simulink model "RL_Vdc_thy"  (R2020b)
settings: Solver=VariableStepAuto  StartTime=0.0  StopTime=0.02  RelTol=1e-3
undefined symbols (not defined in the file): Angle, Magnitude
libraries: powerlib x13, powerlib_meascontrol x3
settings Model: Creator=SAN  LastModifiedBy=macbook
settings DataIOCC: ReturnWorkspaceOutputs=off
settings DebuggingCC: ArithmeticOperatorsInVariantConditions=warning
settings SFSimCC: SimUseLocalCustomCode=off  CustomCodeUndefinedFunction=UseInterfaceOnly
settings RTWCC: RTWUseLocalCustomCode=off

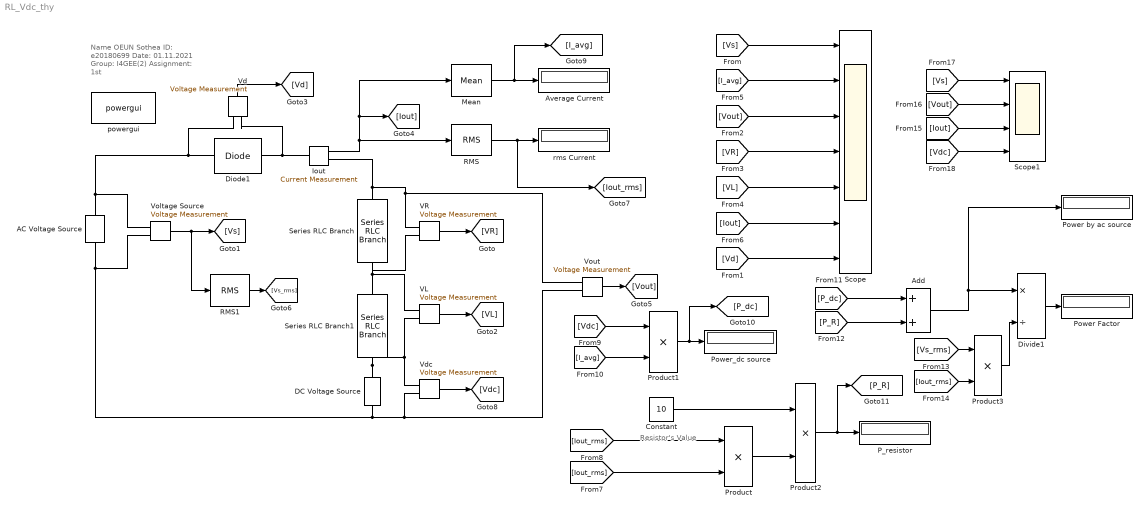
== system RL_Vdc_thy ==
  note: Resistor's Value
  note: Name OEUN Sothea
      | ID: e20180699
      | Date: 01.11.2021
      | Group: I4GEE(2)
      | Assignment: 1st
  " Power by ac source " : Display
  AC Voltage Source : powerlib/Electrical Sources/AC Voltage Source  Amplitude=120*sqrt(2)  Phase=0  Frequency=60  SampleTime=0  Measurements=None  BusType=swing  Pref=10e3  Qref=0  Qmin=-inf  Qmax=+inf
  Add : Sum
  Average Current : Display
  Constant : Constant  Value=10  SampleTime=0
  DC Voltage Source : powerlib/Electrical Sources/DC Voltage Source  Amplitude=100  Measurements=None
  Diode1 : powerlib/Power Electronics/Diode  Ron=0.001  Lon=0  Vf=0.8  IC=0  UseSnubber=0  Rs=500  Cs=250e-9  Measurements=off
  Divide1 : Product  Inputs=*/
  Iout : powerlib/Measurements/Current Measurement  PhasorSimulation=off  OutputType=Magnitude  PSBequivalent=0
  Mean : powerlib_meascontrol/Measurements/Mean  Freq=60  Vinit=0  Ts=0
  P_resistor : Display
  "Power Factor " : Display
  Power_dc source : Display
  Product{,1..3} (4 alike) : Product
  RMS : powerlib_meascontrol/Measurements/RMS  TrueRMS=on  Freq=60  RMSInit=120  Ts=0
  RMS1 : powerlib_meascontrol/Measurements/RMS  TrueRMS=on  Freq=60  RMSInit=120  Ts=0
  Scope : Scope  NumInputPorts=7
  Scope1 : Scope  NumInputPorts=4
  Series RLC Branch : powerlib/Elements/Series RLC Branch  LConnTagsString=__new0  RConnTagsString=__new0  BranchType=R  Resistance=10  Inductance=0.1  SetiL0=off  InitialCurrent=0  Capacitance=1e-6  Setx0=off  InitialVoltage=0  Measurements=None
  Series RLC Branch1 : powerlib/Elements/Series RLC Branch  LConnTagsString=__new0  RConnTagsString=__new0  BranchType=L  Resistance=100  Inductance=0.075  SetiL0=off  InitialCurrent=0  Capacitance=1e-6  Setx0=off  InitialVoltage=0  Measurements=None
  VL : powerlib/Measurements/Voltage Measurement  PhasorSimulation=off  OutputType=Magnitude-Angle  PSBequivalent=0
  "VR " : powerlib/Measurements/Voltage Measurement  PhasorSimulation=off  OutputType=Complex  PSBequivalent=0
  Vd : powerlib/Measurements/Voltage Measurement  PhasorSimulation=off  OutputType=Complex  PSBequivalent=0
  Vdc : powerlib/Measurements/Voltage Measurement  PhasorSimulation=off  OutputType=Magnitude-Angle  PSBequivalent=0
  "Voltage Source " : powerlib/Measurements/Voltage Measurement  PhasorSimulation=off  OutputType=Complex  PSBequivalent=0
  "Vout " : powerlib/Measurements/Voltage Measurement  PhasorSimulation=off  OutputType=Magnitude-Angle  PSBequivalent=0
  powergui : powerlib/powergui  Priority=1  SimulationMode=Continuous  SampleTime=50e-6  frequency=60  Iterations=50  frequencyindice=60  Pbase=100e6  ErrMax=1e-4  UnitsV=kV  UnitsW=MW  buscounter=0  FunctionMessages=off  echomessages=off  EnableUseOfTLC=off  CurrentSourceSwitches=off  DisableSnubberDevices=off  DisableRonSwitches=off  DisableVfSwitches=off  DisplayEquations=off  AutomaticDiscreteSolvers=off  SolverType=Tustin/Backward Euler (TBE)  Interpol=off  ExternalGateDelay=off  methode=off  Ts=100  x0status=blocks  SPID=on  SwTol=0  HookPort=off  NonlinearTolerance=1e-4  nMaxIteration=100  ContinueOnMaxIteration=off  RestoreLinks=warning  ResistiveCurrentMeasurement=off  Frange=[0:2:500]  Ylog=off  Xlog=on  ShowGrid=off  save=off  variable=ZData  structure=0  ZoomFFT=off  StartTime=0.0  cycles=1  DisplayStyle=1  fundamental=60  FreqAxis=off  MaxFrequency=1000  frequencyindicesteady=1  RmsSteady=1  display=off
  rms Current : Display
  wires:
  "Voltage Source "/1 -> RMS1/1, [Vs]
  VL/1 -> [VL]
  Vd/1 -> [Vd]
  "Vout "/1 -> [Vout]
  [Vs] -> Scope/1
  [Vout] -> Scope/3
  [VR] -> Scope/4
  [VL] -> Scope/5
  [Iout] -> Scope/6
  "VR "/1 -> [VR]
  Iout/1 -> RMS/1, [Iout], Mean/1
  Mean/1 -> [I_avg], Average Current/1
  RMS/1 -> [Iout_rms], rms Current/1
  RMS1/1 -> [Vs_rms]
  [Iout_rms] -> Product/1
  [Iout_rms] -> Product/2
  [Vdc] -> Product1/1
  Vdc/1 -> [Vdc]
  [I_avg] -> Product1/2
  Product1/1 -> [P_dc], Power_dc source/1
  Product/1 -> Product2/2
  Product2/1 -> [P_R], P_resistor/1
  Constant/1 -> Product2/1
  [P_dc] -> Add/1
  [P_R] -> Add/2
  Add/1 -> Divide1/1, " Power by ac source "/1
  Product3/1 -> Divide1/2
  Divide1/1 -> "Power Factor "/1
  [Vs_rms] -> Product3/1
  [Iout_rms] -> Product3/2
  [I_avg] -> Scope/2
  [Vd] -> Scope/7
  [Vout] -> Scope1/2
  [Iout] -> Scope1/3
  [Vs] -> Scope1/1
  [Vdc] -> Scope1/4
  connections:
  AC Voltage Source/RConn1 -- "Voltage Source "/LConn1 -- Vd/LConn1 -- Diode1/LConn1
  "Voltage Source "/LConn2 -- Vdc/LConn2 -- "Vout "/LConn2 -- DC Voltage Source/LConn1 -- AC Voltage Source/LConn1
  Iout/LConn1 -- Vd/LConn2 -- Diode1/RConn1
  Iout/RConn1 -- "Vout "/LConn1 -- "VR "/LConn1 -- Series RLC Branch/LConn1
  Series RLC Branch1/LConn1 -- VL/LConn1 -- "VR "/LConn2 -- Series RLC Branch/RConn1
  Series RLC Branch1/RConn1 -- DC Voltage Source/RConn1 -- VL/LConn2 -- Vdc/LConn1
